simulink model "koen_pmsm_current_loop_model"  (R2024b)
settings: Solver=FixedStepDiscrete  StartTime=0.0  StopTime=0.05  FixedStep=6.25e-05  RelTol=1e-3
PreLoadFcn:
  | Ts=6.25e-05; Rs=0.53; Ld=0.0006; Lq=0.0006; psi_f=0.0078; pole_pairs=4; Vdc=24; Vmax=12; Kp_id=2; Ki_id=100; Kp_iq=2; Ki_iq=100; FOC_VD_CMD_SIGN=-1; FOC_VQ_CMD_SIGN=-1; wm=94.24777961; id_ref=0; iq_ref=1; TL=0;
undefined symbols (not defined in the file or in its folder): DiscIntNeverNeededParam
settings Model: Creator=10095  LastModifiedBy=10095

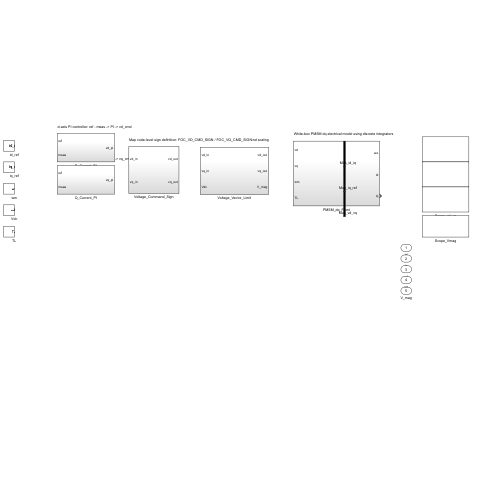
[thumbnail: Simulink's stored preview of the top-level diagram]
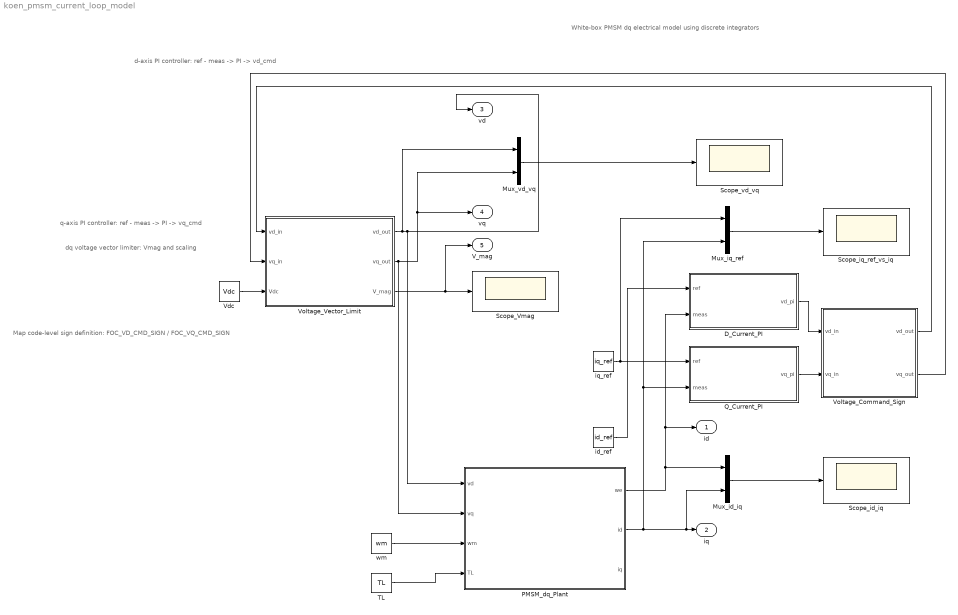
== system koen_pmsm_current_loop_model ==
  note: d-axis PI controller: ref - meas -> PI -> vd_cmd
  note: q-axis PI controller: ref - meas -> PI -> vq_cmd
  note: Map code-level sign definition: FOC_VD_CMD_SIGN / FOC_VQ_CMD_SIGN
  note: dq voltage vector limiter: Vmag and scaling
  note: White-box PMSM dq electrical model using discrete integrators
  D_Current_PI : Subsystem  Description=d-axis PI controller: ref - meas -> PI -> vd_cmd
  Mux_id_iq : Mux  Inputs=2
  Mux_iq_ref : Mux  Inputs=2
  Mux_vd_vq : Mux  Inputs=2
  PMSM_dq_Plant : Subsystem  Description=White-box PMSM dq electrical model using discrete integrators
  Q_Current_PI : Subsystem  Description=q-axis PI controller: ref - meas -> PI -> vq_cmd
  Scope_Vmag : Scope
  Scope_id_iq : Scope
  Scope_iq_ref_vs_iq : Scope
  Scope_vd_vq : Scope
  TL : Constant  Value=TL
  Vdc : Constant  Value=Vdc
  Voltage_Command_Sign : Subsystem  Description=Map code-level sign definition: FOC_VD_CMD_SIGN / FOC_VQ_CMD_SIGN
  Voltage_Vector_Limit : Subsystem  Description=dq voltage vector limiter: Vmag and scaling
  id_ref : Constant  Value=id_ref
  iq_ref : Constant  Value=iq_ref
  wm : Constant  Value=wm
  id : Outport
  iq : Outport  Port=2
  vd : Outport  Port=3
  vq : Outport  Port=4
  V_mag : Outport  Port=5
  wires:
  TL/1 -> PMSM_dq_Plant/4(TL)
  Vdc/1 -> Voltage_Vector_Limit/3(Vdc)
  iq_ref/1 -> Q_Current_PI/1(ref), Mux_iq_ref/1
  id_ref/1 -> D_Current_PI/1(ref)
  Voltage_Vector_Limit/1(vd_out) -> PMSM_dq_Plant/1(vd), vd/1, Mux_vd_vq/1
  wm/1 -> PMSM_dq_Plant/3(wm)
  Voltage_Vector_Limit/3(V_mag) -> Scope_Vmag/1, V_mag/1
  Voltage_Vector_Limit/2(vq_out) -> Mux_vd_vq/2, vq/1, PMSM_dq_Plant/2(vq)
  Mux_vd_vq/1 -> Scope_vd_vq/1
  PMSM_dq_Plant/1(we) -> D_Current_PI/2(meas), id/1, Mux_id_iq/1
  PMSM_dq_Plant/2(id) -> Mux_id_iq/2, iq/1, Q_Current_PI/2(meas), Mux_iq_ref/2
  Mux_iq_ref/1 -> Scope_iq_ref_vs_iq/1
  D_Current_PI/1(vd_pi) -> Voltage_Command_Sign/1(vd_in)
  Q_Current_PI/1(vq_pi) -> Voltage_Command_Sign/2(vq_in)
  Mux_id_iq/1 -> Scope_id_iq/1
  Voltage_Command_Sign/1(vd_out) -> Voltage_Vector_Limit/1(vd_in)
  Voltage_Command_Sign/2(vq_out) -> Voltage_Vector_Limit/2(vq_in)

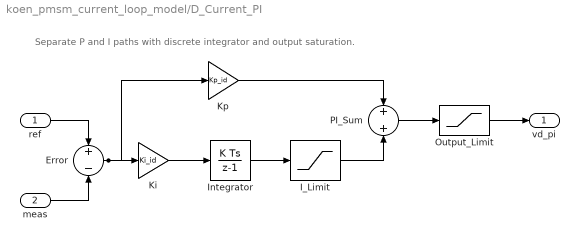
== system koen_pmsm_current_loop_model/D_Current_PI ==
  note: Separate P and I paths with discrete integrator and output saturation.
  ref : Inport
  meas : Inport  Port=2
  Error : Sum  Inputs=+-
  I_Limit : Saturate  UpperLimit=20  LowerLimit=-20
  Integrator : DiscreteIntegrator  SampleTime=Ts  ICPrevOutput=DiscIntNeverNeededParam  ICPrevScaledInput=DiscIntNeverNeededParam
  Ki : Gain  Gain=Ki_id
  Kp : Gain  Gain=Kp_id
  Output_Limit : Saturate  UpperLimit=15  LowerLimit=-15
  PI_Sum : Sum
  vd_pi : Outport
  wires:
  ref/1 -> Error/1
  Kp/1 -> PI_Sum/1
  Ki/1 -> Integrator/1
  Error/1 -> Kp/1, Ki/1
  meas/1 -> Error/2
  Integrator/1 -> I_Limit/1
  I_Limit/1 -> PI_Sum/2
  PI_Sum/1 -> Output_Limit/1
  Output_Limit/1 -> vd_pi/1

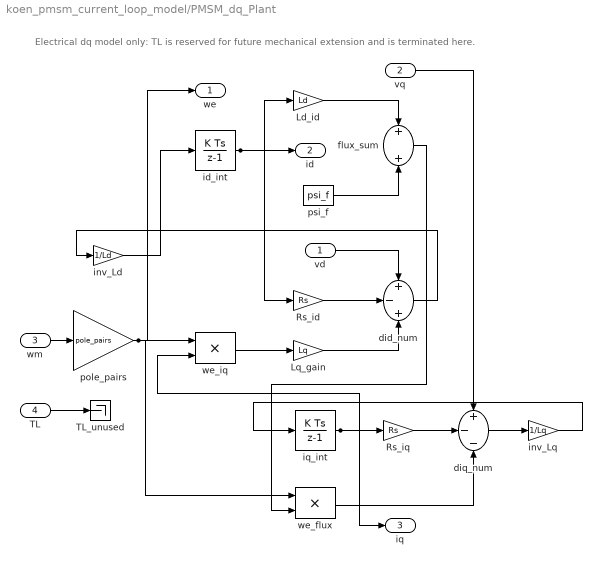
== system koen_pmsm_current_loop_model/PMSM_dq_Plant ==
  note: Electrical dq model only: TL is reserved for future mechanical extension and is terminated here.
  vd : Inport
  vq : Inport  Port=2
  wm : Inport  Port=3
  TL : Inport  Port=4
  Ld_id : Gain  Gain=Ld
  Lq_gain : Gain  Gain=Lq
  Rs_id : Gain  Gain=Rs
  Rs_iq : Gain  Gain=Rs
  TL_unused : Terminator
  did_num : Sum  Inputs=+-+
  diq_num : Sum  Inputs=+--
  flux_sum : Sum
  id_int : DiscreteIntegrator  SampleTime=Ts  ICPrevOutput=DiscIntNeverNeededParam  ICPrevScaledInput=DiscIntNeverNeededParam
  inv_Ld : Gain  Gain=1/Ld
  inv_Lq : Gain  Gain=1/Lq
  iq_int : DiscreteIntegrator  SampleTime=Ts  ICPrevOutput=DiscIntNeverNeededParam  ICPrevScaledInput=DiscIntNeverNeededParam
  pole_pairs : Gain  Gain=pole_pairs
  psi_f : Constant  Value=psi_f
  we_flux : Product
  we_iq : Product
  we : Outport
  id : Outport  Port=2
  iq : Outport  Port=3
  wires:
  wm/1 -> pole_pairs/1
  TL/1 -> TL_unused/1
  pole_pairs/1 -> we_flux/1, we/1, we_iq/1
  inv_Lq/1 -> iq_int/1
  we_flux/1 -> diq_num/3
  inv_Ld/1 -> id_int/1
  psi_f/1 -> flux_sum/2
  Ld_id/1 -> flux_sum/1
  vd/1 -> did_num/1
  id_int/1 -> Rs_id/1, id/1, Ld_id/1
  we_iq/1 -> Lq_gain/1
  Rs_id/1 -> did_num/2
  iq_int/1 -> we_iq/2, iq/1, Rs_iq/1
  Lq_gain/1 -> did_num/3
  vq/1 -> diq_num/1
  diq_num/1 -> inv_Lq/1
  flux_sum/1 -> we_flux/2
  did_num/1 -> inv_Ld/1
  Rs_iq/1 -> diq_num/2

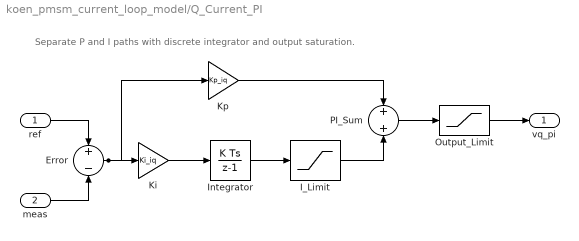
== system koen_pmsm_current_loop_model/Q_Current_PI ==
  note: Separate P and I paths with discrete integrator and output saturation.
  ref : Inport
  meas : Inport  Port=2
  Error : Sum  Inputs=+-
  I_Limit : Saturate  UpperLimit=20  LowerLimit=-20
  Integrator : DiscreteIntegrator  SampleTime=Ts  ICPrevOutput=DiscIntNeverNeededParam  ICPrevScaledInput=DiscIntNeverNeededParam
  Ki : Gain  Gain=Ki_iq
  Kp : Gain  Gain=Kp_iq
  Output_Limit : Saturate  UpperLimit=15  LowerLimit=-15
  PI_Sum : Sum
  vq_pi : Outport
  wires:
  meas/1 -> Error/2
  ref/1 -> Error/1
  Kp/1 -> PI_Sum/1
  Error/1 -> Kp/1, Ki/1
  I_Limit/1 -> PI_Sum/2
  PI_Sum/1 -> Output_Limit/1
  Integrator/1 -> I_Limit/1
  Ki/1 -> Integrator/1
  Output_Limit/1 -> vq_pi/1

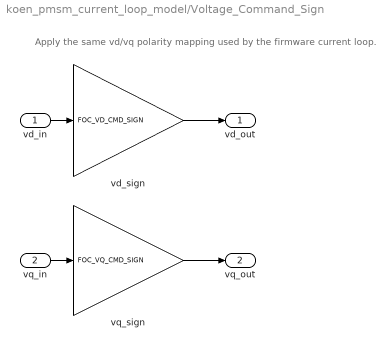
== system koen_pmsm_current_loop_model/Voltage_Command_Sign ==
  note: Apply the same vd/vq polarity mapping used by the firmware current loop.
  vd_in : Inport
  vq_in : Inport  Port=2
  vd_sign : Gain  Gain=FOC_VD_CMD_SIGN
  vq_sign : Gain  Gain=FOC_VQ_CMD_SIGN
  vd_out : Outport
  vq_out : Outport  Port=2
  wires:
  vd_in/1 -> vd_sign/1
  vq_in/1 -> vq_sign/1
  vd_sign/1 -> vd_out/1
  vq_sign/1 -> vq_out/1

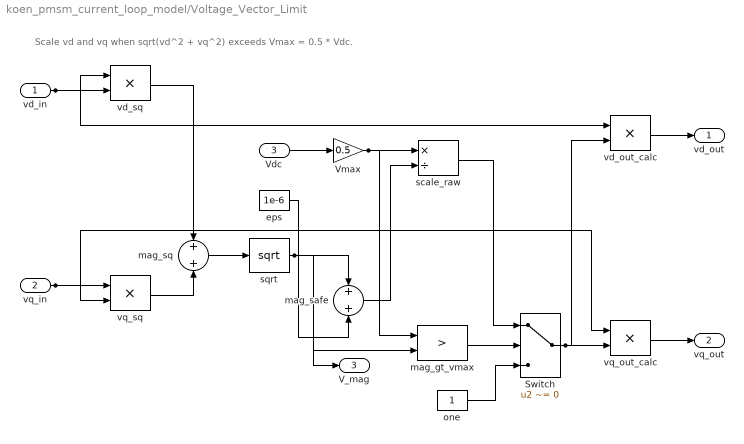
== system koen_pmsm_current_loop_model/Voltage_Vector_Limit ==
  note: Scale vd and vq when sqrt(vd^2 + vq^2) exceeds Vmax = 0.5 * Vdc.
  vd_in : Inport
  vq_in : Inport  Port=2
  Vdc : Inport  Port=3
  Switch : Switch  Criteria=u2 ~= 0  Threshold=0.5  SaturateOnIntegerOverflow=off  InputSameDT=off
  Vmax : Gain  Gain=0.5
  eps : Constant  Value=1e-6
  mag_gt_vmax : RelationalOperator  Operator=>  OutDataTypeStr=boolean  RndMeth=Simplest  InputSameDT=off
  mag_safe : Sum
  mag_sq : Sum
  one : Constant
  scale_raw : Product  Inputs=*/
  sqrt : Math  Operator=sqrt
  vd_out_calc : Product
  vd_sq : Product
  vq_out_calc : Product
  vq_sq : Product
  vd_out : Outport
  vq_out : Outport  Port=2
  V_mag : Outport  Port=3
  wires:
  vq_in/1 -> vq_out_calc/1, vq_sq/2, vq_sq/1
  vd_in/1 -> vd_out_calc/1, vd_sq/1, vd_sq/2
  Vdc/1 -> Vmax/1
  sqrt/1 -> mag_gt_vmax/2, mag_safe/1, V_mag/1
  eps/1 -> mag_safe/2
  vd_sq/1 -> mag_sq/1
  mag_sq/1 -> sqrt/1
  vq_sq/1 -> mag_sq/2
  Vmax/1 -> mag_gt_vmax/1, scale_raw/1
  mag_safe/1 -> scale_raw/2
  mag_gt_vmax/1 -> Switch/2
  scale_raw/1 -> Switch/1
  one/1 -> Switch/3
  vq_out_calc/1 -> vq_out/1
  Switch/1 -> vd_out_calc/2, vq_out_calc/2
  vd_out_calc/1 -> vd_out/1
